simulink model "model"  (R2013b)
settings: Solver=ode3  StartTime=0.0  StopTime=10.0  FixedStep=0.01  RelTol=1e-3
libraries: simulink x1
settings Model: Creator=Sander  LastModifiedBy=Sander
settings ConfigurationSet: Description=SimMechanics 2G

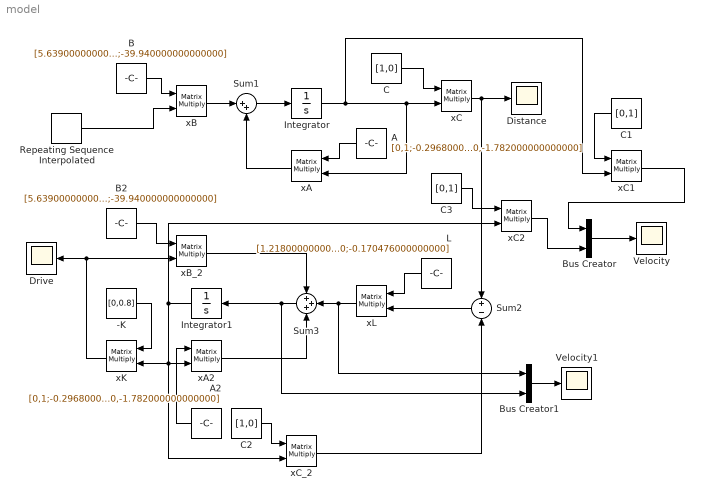
== system model ==
  -K : Constant  Value=[0,0.8]  VectorParams1D=off
  A : Constant  Value=[0,1;-0.296800000000000,-1.782000000000000]  VectorParams1D=off
  A2 : Constant  Value=[0,1;-0.296800000000000,-1.782000000000000]  VectorParams1D=off
  B : Constant  Value=[5.639000000000000;-39.940000000000000]  VectorParams1D=off
  B2 : Constant  Value=[5.639000000000000;-39.940000000000000]  VectorParams1D=off
  Bus Creator : BusCreator  Inputs=2
  Bus Creator1 : BusCreator  Inputs=2
  C : Constant  Value=[1,0]  VectorParams1D=off
  C1 : Constant  Value=[0,1]  VectorParams1D=off
  C2 : Constant  Value=[1,0]  VectorParams1D=off
  C3 : Constant  Value=[0,1]  VectorParams1D=off
  Distance : Scope
      settings: TimeRange=10  YMin=2.2872  YMax=2.2886
  Drive : Scope
      settings: TimeRange=10  YMin=-1e+61  YMax=0
  Integrator : Integrator  InitialCondition=[3;-3]
  Integrator1 : Integrator  InitialCondition=[3;-3]
  L : Constant  Value=[1.218000000000000;-0.170476000000000]  VectorParams1D=off
  Repeating Sequence Interpolated : simulink/Sources/Repeating Sequence Interpolated  OutValues=[0 0.3 0.1 0.4 0.2 0.1 0.1].'  TimeValues=[0 0.1 0.5 0.6 0.8 1 10].'  LookUpMeth=Interpolation-Use End Values  tsamp=0.01  OutMin=[]  OutMax=[]  OutDataTypeStr=double  OutputDataTypeScalingMode=double  OutDataType=fixdt(0,8)  OutScaling=2^-10
  Sum1 : Sum  Inputs=|++
  Sum2 : Sum  Inputs=+|-
  Sum3 : Sum  Inputs=+++
  Velocity : Scope
      settings: TimeRange=10  YMin=2.2872  YMax=2.2886  SaveName=ScopeData2
  Velocity1 : Scope
      settings: TimeRange=10  YMin=2.2872  YMax=2.2886  SaveName=ScopeData3
  xA : Product  Multiplication=Matrix(*)
  xA2 : Product  Multiplication=Matrix(*)
  xB : Product  Multiplication=Matrix(*)
  xB_2 : Product  Multiplication=Matrix(*)
  xC : Product  Multiplication=Matrix(*)
  xC1 : Product  Multiplication=Matrix(*)
  xC2 : Product  Multiplication=Matrix(*)
  xC_2 : Product  Multiplication=Matrix(*)
  xK : Product  Multiplication=Matrix(*)
  xL : Product  Multiplication=Matrix(*)
  wires:
  B/1 -> xB/1
  xK/1 -> xB_2/2, Drive/1
  A/1 -> xA/1
  Sum1/1 -> Integrator/1
  xA/1 -> Sum1/2
  xB/1 -> Sum1/1
  C/1 -> xC/1
  xC/1 -> Sum2/1, Distance/1
  Sum2/1 -> xL/2
  L/1 -> xL/1
  Sum3/1 -> Bus Creator1/2, Integrator1/1
  C2/1 -> xC_2/1
  xC_2/1 -> Sum2/2
  xB_2/1 -> Sum3/1
  A2/1 -> xA2/1
  xA2/1 -> Sum3/3
  Integrator/1 -> xC1/2, xA/2, xC/2
  B2/1 -> xB_2/1
  -K/1 -> xK/1
  Bus Creator/1 -> Velocity/1
  C1/1 -> xC1/1
  xC1/1 -> Bus Creator/1
  xC2/1 -> Bus Creator/2
  C3/1 -> xC2/1
  Integrator1/1 -> xC2/2, xK/2, xC_2/2, xA2/2
  xL/1 -> Bus Creator1/1, Sum3/2
  Repeating Sequence Interpolated/1 -> xB/2
  Bus Creator1/1 -> Velocity1/1
